simulink model "basic_model_hodgklin_huxley"  (R2021a)
settings: Solver=FixedStepAuto  StartTime=0.0  StopTime=30e3  FixedStep=30e-6  RelTol=1e-3
settings Model: Creator=Bremdows  LastModifiedBy=Bremdows

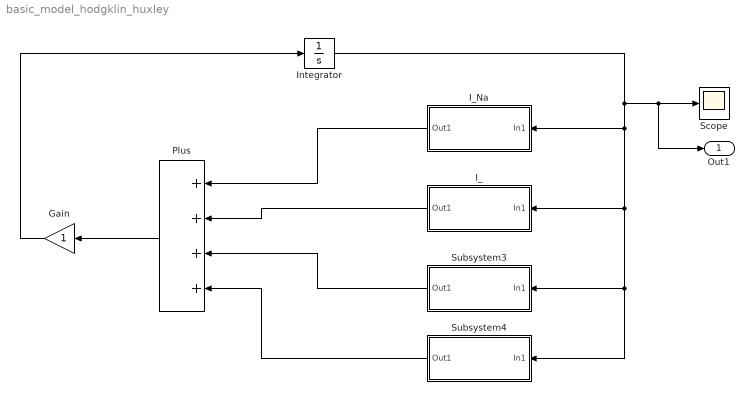
== system basic_model_hodgklin_huxley ==
  Gain : Gain
  I_ : Subsystem
  I_Na : Subsystem
  Integrator : Integrator  InitialCondition=-60e3
  Plus : Sum  Inputs=++++
  Scope : Scope
  Subsystem3 : Subsystem
  Subsystem4 : Subsystem
  Out1 : Outport
  wires:
  I_Na/1(Out1) -> Plus/1
  I_/1(Out1) -> Plus/2
  Subsystem3/1(Out1) -> Plus/3
  Subsystem4/1(Out1) -> Plus/4
  Plus/1 -> Gain/1
  Gain/1 -> Integrator/1
  Integrator/1 -> Scope/1, Out1/1, I_/1(In1), Subsystem3/1(In1), Subsystem4/1(In1), I_Na/1(In1)

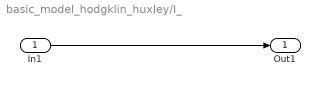
== system basic_model_hodgklin_huxley/I_ ==
  In1 : Inport
  Out1 : Outport
  wires:
  In1/1 -> Out1/1

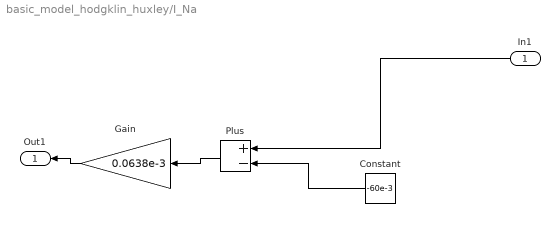
== system basic_model_hodgklin_huxley/I_Na ==
  In1 : Inport
  Constant : Constant  Value=-60e-3
  Gain : Gain  Gain=0.0638e-3
  Plus : Sum  Inputs=+-
  Out1 : Outport
  wires:
  In1/1 -> Plus/1
  Gain/1 -> Out1/1
  Plus/1 -> Gain/1
  Constant/1 -> Plus/2

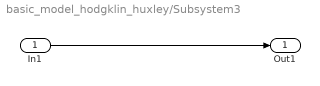
== system basic_model_hodgklin_huxley/Subsystem3 ==
  In1 : Inport
  Out1 : Outport
  wires:
  In1/1 -> Out1/1

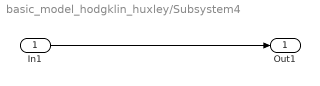
== system basic_model_hodgklin_huxley/Subsystem4 ==
  In1 : Inport
  Out1 : Outport
  wires:
  In1/1 -> Out1/1
